simulink model "sampleModel1506"  (R2023a)
settings: Solver=VariableStepAuto  StartTime=0.0  StopTime=10.0  RelTol=1e-3
libraries: hdlsllib x5, simulink x3
settings Model: Creator=user1  LastModifiedBy=user1

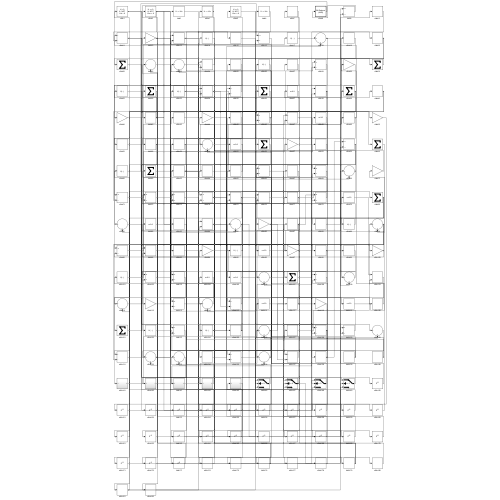
[thumbnail: Simulink's stored preview of the top-level diagram]
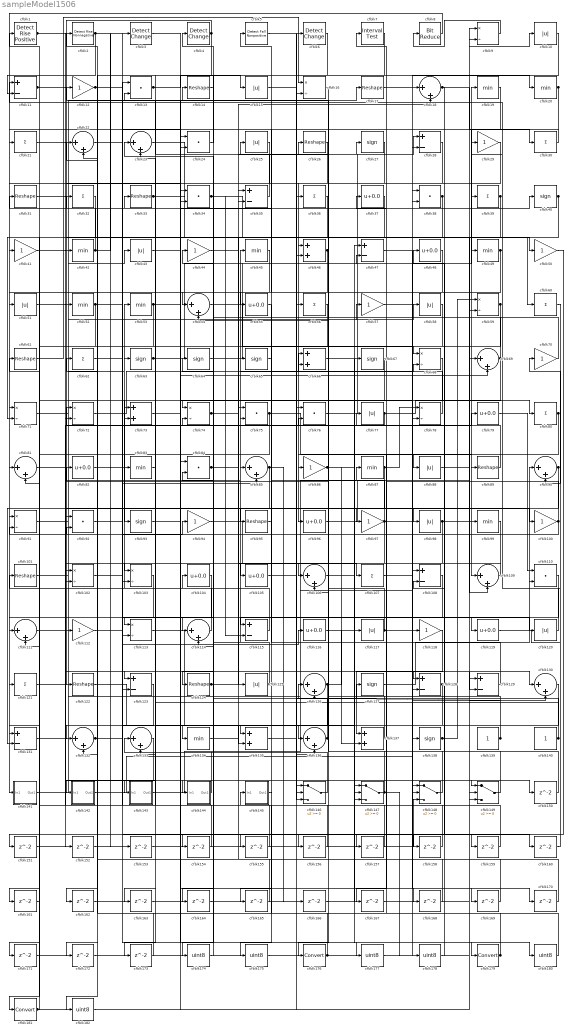
== system sampleModel1506 ==
  cfblk1 : hdlsllib/Logic and Bit Operations/Detect Rise Positive  vinit=0  OutDataTypeStr=boolean
  cfblk{10,15,25,43,51,58,77,88,98,117,120,125} (12 alike) : Abs  SaturateOnIntegerOverflow=off
  cfblk{12,29,41,44,50,57,70,86,94,97,100,112,118} (13 alike) : Gain
  cfblk{14,17,26,31,33,61,89,95,101,122,124} (11 alike) : Reshape
  cfblk{9,16,59,68,71..72,74,78,91,102..103,113} (12 alike) : Product  Inputs=*/  RndMeth=Zero  SaturateOnIntegerOverflow=on
  cfblk{37,48,55,79,82,96,104..105,116,119} (10 alike) : Bias  Bias=0.0  SaturateOnIntegerOverflow=off
  cfblk{18,22..23,54,69,81,85,90,106,109,111,114,126,130,132..133,136} (17 alike) : Sum  Inputs=|++
  cfblk{21,30,32,36,39,56,60,62,80,107,121} (11 alike) : Sum  Inputs=+
  cfblk{11,28,35,47,108,115,123,128..129,131} (10 alike) : Sum  Inputs=+-
  cfblk{13,24,34,38,75..76,84,92,110} (9 alike) : DotProduct  OutDataTypeStr=Inherit: Inherit via internal rule
  cfblk{27,40,63..65,67,93,127,138} (9 alike) : Signum
  cfblk{19..20,42,45,49,52..53,83,87,99,134} (11 alike) : MinMax
  cfblk{46,66,73,135,137} (5 alike) : Sum
  cfblk139 : Constant  SampleTime=-1
  cfblk140 : Constant  SampleTime=-1
  cfblk141 : Subsystem
      settings: LibrarySourceBlock=|
      | hdlsllib/Ports &
      | Subsystems/Subsystem
  cfblk142 : Subsystem
      settings: LibrarySourceBlock=|
      | hdlsllib/Ports &
      | Subsystems/Subsystem
  cfblk143 : Subsystem
      settings: LibrarySourceBlock=|
      | hdlsllib/Ports &
      | Subsystems/Subsystem
  cfblk144 : Subsystem
      settings: LibrarySourceBlock=|
      | hdlsllib/Ports &
      | Subsystems/Subsystem
  cfblk145 : Subsystem
      settings: LibrarySourceBlock=|
      | hdlsllib/Ports &
      | Subsystems/Subsystem
  cfblk{146..149} (4 alike) : Switch  SaturateOnIntegerOverflow=off  InputSameDT=off
  cfblk{150..173} (24 alike) : Delay  SampleTime=1
  cfblk{174..175,177..178,180,182} (6 alike) : DataTypeConversion  OutDataTypeStr=uint8  SaturateOnIntegerOverflow=off  RndMeth=Floor
  cfblk176 : DataTypeConversion  SaturateOnIntegerOverflow=off  RndMeth=Floor
  cfblk179 : DataTypeConversion  SaturateOnIntegerOverflow=off  RndMeth=Floor
  cfblk181 : DataTypeConversion  SaturateOnIntegerOverflow=off  RndMeth=Floor
  cfblk2 : hdlsllib/Logic and Bit Operations/Detect Rise Nonnegative  vinit=0  OutDataTypeStr=boolean
  cfblk3 : simulink/Logic and Bit Operations/Detect Change  vinit=0  OutDataTypeStr=boolean
      settings: LibrarySourceBlock=|
      | hdlsllib/Logic and Bit
      | Operations/Detect
      | Change
  cfblk4 : simulink/Logic and Bit Operations/Detect Change  vinit=0  OutDataTypeStr=boolean
      settings: LibrarySourceBlock=|
      | hdlsllib/Logic and Bit
      | Operations/Detect
      | Change
  cfblk5 : hdlsllib/Logic and Bit Operations/Detect Fall Nonpositive  vinit=0  OutDataTypeStr=boolean
  cfblk6 : simulink/Logic and Bit Operations/Detect Change  vinit=0  OutDataTypeStr=boolean
      settings: LibrarySourceBlock=|
      | hdlsllib/Logic and Bit
      | Operations/Detect
      | Change
  cfblk7 : hdlsllib/Logic and Bit Operations/Interval Test  IntervalClosedRight=on  uplimit=0.5  IntervalClosedLeft=on  lowlimit=-0.5  OutDataTypeStr=boolean
  cfblk8 : hdlsllib/Logic and Bit Operations/Bit Reduce  mode=AND
  wires:
  cfblk19/1 -> cfblk109/1
  cfblk125/1 -> cfblk45/1, cfblk92/2
  cfblk65/1 -> cfblk33/1
  cfblk131/1 -> cfblk43/1
  cfblk42/1 -> cfblk3/1, cfblk31/1, cfblk153/1
  cfblk126/1 -> cfblk117/1, cfblk146/3
  cfblk144/1(Out1) -> cfblk133/1
  cfblk75/1 -> cfblk89/1, cfblk91/1
  cfblk118/1 -> cfblk137/1
  cfblk147/1 -> cfblk44/1, cfblk178/1
  cfblk4/1 -> cfblk122/1, cfblk132/2
  cfblk91/1 -> cfblk14/1
  cfblk115/1 -> cfblk53/1
  cfblk110/1 -> cfblk115/1
  cfblk94/1 -> cfblk107/1
  cfblk61/1 -> cfblk16/1
  cfblk98/1 -> cfblk112/1, cfblk109/2
  cfblk121/1 -> cfblk85/1
  cfblk113/1 -> cfblk135/1
  cfblk23/1 -> cfblk125/1
  cfblk141/1(Out1) -> cfblk87/1
  cfblk2/1 -> cfblk135/2, cfblk83/1, cfblk11/2, cfblk24/2
  cfblk67/1 -> cfblk93/1
  cfblk64/1 -> cfblk19/1
  cfblk139/1 -> cfblk134/1, cfblk126/2, cfblk54/2
  cfblk77/1 -> cfblk80/1, cfblk76/2
  cfblk43/1 -> cfblk17/1
  cfblk44/1 -> cfblk106/1
  cfblk117/1 -> cfblk65/1, cfblk169/1
  cfblk47/1 -> cfblk138/1
  cfblk119/1 -> cfblk70/1
  cfblk10/1 -> cfblk113/1
  cfblk80/1 -> cfblk156/1, cfblk157/1, cfblk158/1
  cfblk45/1 -> cfblk52/1
  cfblk134/1 -> cfblk27/1
  cfblk54/1 -> cfblk118/1
  cfblk34/1 -> cfblk99/1, cfblk115/2
  cfblk52/1 -> cfblk95/1, cfblk72/2
  cfblk107/1 -> cfblk38/1
  cfblk71/1 -> cfblk58/1
  cfblk111/1 -> cfblk79/1
  cfblk8/1 -> cfblk141/1(In1)
  cfblk26/1 -> cfblk96/1
  cfblk25/1 -> cfblk42/1
  cfblk127/1 -> cfblk90/1
  cfblk106/1 -> cfblk119/1
  cfblk124/1 -> cfblk39/1, cfblk18/2
  cfblk88/1 -> cfblk10/1
  cfblk143/1(Out1) -> cfblk18/1
  cfblk129/1 -> cfblk75/2
  cfblk148/1 -> cfblk25/1
  cfblk79/1 -> cfblk110/1
  cfblk76/1 -> cfblk28/1
  cfblk122/1 -> cfblk147/1
  cfblk87/1 -> cfblk78/1, cfblk171/1, cfblk172/1
  cfblk101/1 -> cfblk63/1
  cfblk5/1 -> cfblk56/1
  cfblk62/1 -> cfblk179/1
  cfblk48/1 -> cfblk81/1
  cfblk35/1 -> cfblk12/1
  cfblk104/1 -> cfblk133/2
  cfblk138/1 -> cfblk48/1, cfblk59/1
  cfblk29/1 -> cfblk71/1
  cfblk149/1 -> cfblk13/2
  cfblk16/1 -> cfblk86/1
  cfblk109/1 -> cfblk105/1
  cfblk70/1 -> cfblk23/1
  cfblk69/1 -> cfblk32/1, cfblk111/1
  cfblk14/1 -> cfblk124/1
  cfblk24/1 -> cfblk4/1
  cfblk27/1 -> cfblk46/1
  cfblk92/1 -> cfblk77/1
  cfblk51/1 -> cfblk144/1(In1)
  cfblk18/1 -> cfblk68/1, cfblk30/1
  cfblk72/1 -> cfblk68/2
  cfblk137/1 -> cfblk82/1
  cfblk105/1 -> cfblk128/1
  cfblk11/1 -> cfblk100/1, cfblk146/2
  cfblk46/1 -> cfblk103/1, cfblk26/1
  cfblk95/1 -> cfblk5/1
  cfblk81/1 -> cfblk149/1
  cfblk99/1 -> cfblk128/2
  cfblk39/1 -> cfblk114/1, cfblk88/1
  cfblk12/1 -> cfblk136/2, cfblk150/1, cfblk182/1
  cfblk102/1 -> cfblk85/2
  cfblk36/1 -> cfblk181/1
  cfblk57/1 -> cfblk49/1
  cfblk3/1 -> cfblk50/1
  cfblk103/1 -> cfblk121/1
  cfblk116/1 -> cfblk67/1
  cfblk1/1 -> cfblk129/2, cfblk34/2
  cfblk63/1 -> cfblk28/2, cfblk69/2, cfblk40/1
  cfblk146/1 -> cfblk73/1
  cfblk97/1 -> cfblk136/1, cfblk130/2, cfblk72/1
  cfblk41/1 -> cfblk123/1
  cfblk78/1 -> cfblk66/1
  cfblk32/1 -> cfblk71/2
  cfblk142/1(Out1) -> cfblk38/2
  cfblk130/1 -> cfblk148/2
  cfblk135/1 -> cfblk127/1
  cfblk108/1 -> cfblk176/1
  cfblk136/1 -> cfblk106/2, cfblk126/1
  cfblk28/1 -> cfblk41/1
  cfblk9/1 -> cfblk8/1
  cfblk128/1 -> cfblk163/1, cfblk164/1
  cfblk123/1 -> cfblk132/1
  cfblk132/1 -> cfblk94/1, cfblk116/1
  cfblk85/1 -> cfblk142/1(In1), cfblk166/1
  cfblk114/1 -> cfblk101/1
  cfblk89/1 -> cfblk22/2
  cfblk40/1 -> cfblk102/1, cfblk51/1
  cfblk100/1 -> cfblk37/1, cfblk91/2
  cfblk13/1 -> cfblk15/1, cfblk97/1
  cfblk38/1 -> cfblk54/1, cfblk111/2
  cfblk86/1 -> cfblk137/2, cfblk180/1
  cfblk37/1 -> cfblk74/1
  cfblk59/1 -> cfblk143/1(In1), cfblk103/2
  cfblk58/1 -> cfblk102/2
  cfblk74/1 -> cfblk35/2, cfblk98/1
  cfblk53/1 -> cfblk160/1, cfblk161/1
  cfblk60/1 -> cfblk90/2
  cfblk84/1 -> cfblk130/1, cfblk47/2
  cfblk20/1 -> cfblk55/1, cfblk114/2
  cfblk21/1 -> cfblk46/2
  cfblk96/1 -> cfblk9/2
  cfblk15/1 -> cfblk147/3
  cfblk49/1 -> cfblk123/2, cfblk29/1
  cfblk30/1 -> cfblk21/1
  cfblk90/1 -> cfblk131/1, cfblk131/2, cfblk167/1
  cfblk33/1 -> cfblk60/1, cfblk78/2
  cfblk7/1 -> cfblk113/2
  cfblk22/1 -> cfblk120/1
  cfblk140/1 -> cfblk66/2, cfblk73/2
  cfblk120/1 -> cfblk11/1
  cfblk17/1 -> cfblk20/1
  cfblk112/1 -> cfblk57/1
  cfblk150/1 -> cfblk129/1
  cfblk50/1 -> cfblk151/1
  cfblk151/1 -> cfblk16/2
  cfblk31/1 -> cfblk152/1
  cfblk152/1 -> cfblk148/1
  cfblk153/1 -> cfblk148/3
  cfblk56/1 -> cfblk154/1
  cfblk154/1 -> cfblk84/1
  cfblk68/1 -> cfblk155/1
  cfblk155/1 -> cfblk1/1
  cfblk156/1 -> cfblk75/1
  cfblk157/1 -> cfblk92/1
  cfblk158/1 -> cfblk23/2
  cfblk82/1 -> cfblk159/1
  cfblk159/1 -> cfblk13/1
  cfblk160/1 -> cfblk110/2
  cfblk161/1 -> cfblk81/2
  cfblk133/1 -> cfblk162/1
  cfblk162/1 -> cfblk147/2
  cfblk163/1 -> cfblk76/1
  cfblk164/1 -> cfblk74/2
  cfblk55/1 -> cfblk165/1
  cfblk165/1 -> cfblk35/1
  cfblk166/1 -> cfblk69/1
  cfblk167/1 -> cfblk149/3
  cfblk66/1 -> cfblk168/1
  cfblk168/1 -> cfblk22/1
  cfblk169/1 -> cfblk47/1
  cfblk73/1 -> cfblk170/1
  cfblk170/1 -> cfblk146/1
  cfblk171/1 -> cfblk9/1
  cfblk172/1 -> cfblk59/2
  cfblk83/1 -> cfblk173/1
  cfblk173/1 -> cfblk2/1
  cfblk6/1 -> cfblk174/1
  cfblk174/1 -> cfblk104/1
  cfblk145/1(Out1) -> cfblk175/1
  cfblk175/1 -> cfblk6/1
  cfblk176/1 -> cfblk34/1, cfblk145/1(In1)
  cfblk93/1 -> cfblk177/1
  cfblk177/1 -> cfblk108/1
  cfblk178/1 -> cfblk108/2
  cfblk179/1 -> cfblk7/1, cfblk64/1, cfblk84/2
  cfblk180/1 -> cfblk62/1
  cfblk181/1 -> cfblk149/2, cfblk24/1, cfblk61/1
  cfblk182/1 -> cfblk36/1

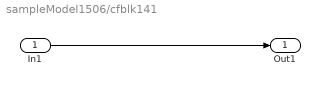
== system sampleModel1506/cfblk141 ==
  In1 : Inport
  Out1 : Outport
  wires:
  In1/1 -> Out1/1

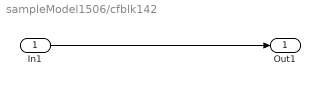
== system sampleModel1506/cfblk142 ==
  In1 : Inport
  Out1 : Outport
  wires:
  In1/1 -> Out1/1

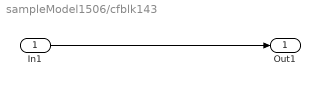
== system sampleModel1506/cfblk143 ==
  In1 : Inport
  Out1 : Outport
  wires:
  In1/1 -> Out1/1

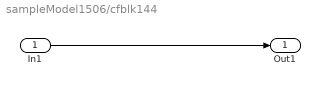
== system sampleModel1506/cfblk144 ==
  In1 : Inport
  Out1 : Outport
  wires:
  In1/1 -> Out1/1

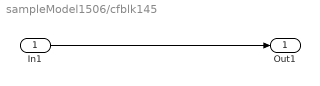
== system sampleModel1506/cfblk145 ==
  In1 : Inport
  Out1 : Outport
  wires:
  In1/1 -> Out1/1
